simulink model "test_layerwall_static"  (R2013b)
settings: Solver=ode45  StartTime=0.0  StopTime=2*24*3600  RelTol=1e-3
libraries: carnot x9
settings Model: Creator=drhf  LastModifiedBy=drhf
settings OptimizationCC: InlineParams=on

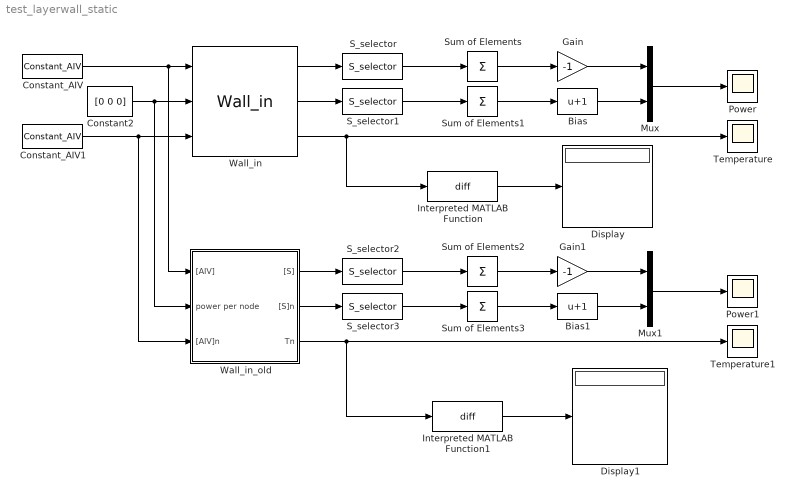
== system test_layerwall_static ==
  Bias : Bias  Bias=1
  Bias1 : Bias  Bias=1
  Constant2 : Constant  Value=[0 0 0]
  Constant_AIV : carnot/Source/Ventilation/Constant_AIV  Tsens=20  Tcon=20  Trad=20  mw=0.012  mco=0.01  rhoair=1.2  cpair=1004  pair=100000  nair=0.5
  Constant_AIV1 : carnot/Source/Ventilation/Constant_AIV  Tsens=0  Tcon=0  Trad=0  mw=0.012  mco=0.01  rhoair=1.2  cpair=1004  pair=100000  nair=0.5
  Display : Display
  Display1 : Display
  Gain : Gain  Gain=-1
  Gain1 : Gain  Gain=-1
  Interpreted MATLAB Function : MATLABFcn  MATLABFcn=diff
  Interpreted MATLAB Function1 : MATLABFcn  MATLABFcn=diff
  Mux : Mux  Inputs=2
  Mux1 : Mux  Inputs=2
  Power : Scope
  Power1 : Scope
      settings: SaveName=ScopeData2
  S_selector{,1..3} (4 alike) : carnot/Outputs/S_selector  e1=off  e2=off  e3=off  e4=off  e5=off  e6=off  e7=on  e8=on  e9=off  e10=off  e11=off  e12=off  e13=off
  Sum of Elements{,1..3} (4 alike) : Sum  Inputs=+
  Temperature : Scope
  Temperature1 : Scope
      settings: SaveName=ScopeData3
  Wall_in : carnot/Load/Houses/wall_floor/Wall_in  wallsize=[10 10]  d=[0.1 0.1 0.1]  cond=[1 1 1]  cwall=[0.28 0.28 0.28]*3600  rho=[2000 200 2000]  emission_in=.96  dactive=[0.075 0.15 0.225]  t0=10  tau=10*3600
  Wall_in_old : Subsystem  AncestorBlock=carnot/Load/Houses/wall_floor/Wall_in  mask(inner wall){wallsize=[10 10], d=[0.1 0.1 0.1], cond=[1 1 1], cwall=[0.28 0.28 0.28]*3600, rho=[2000 200 2000], emission_in=.96, dactive=[0.075 0.15 0.225], t0=10, tau=10*3600}
      mask prompts: wallsize "size of wall [m] [height width]"; d "thickness of layers [m] (vector) (0 = towards this room)"; cond "conductivity of layers [W/(m*K)] (vector)"; cwall "capacity of layers [J/(m³*K)] (vector)"; rho "density of layers [kg/m³]"; emission_in "emission of wall surface"; dactive "depth active layer in m from inner surface  (-1 = none)"; t0 "initial temperature [degree centigrade]"; tau "time-constant of wall [s]"
      mask help:
      | This is the model of an inner wall in a house.
      | first element of the vector = layer to room ([AIV], [S])
      | last element of the vector = layer to neighbour room ([AIV]n, [S]n)
      mask init:
      | position = [0 90 0 ];
      | % nodes = length(d);
      | wallheight = wallsize(1);
      | wallsurface = wallsize(1)*wallsize(2);
      | 
      | if (dactive>=0) 
      |     active = 1;
      | else
      |     active = 0;
      | end
      mask Help: web(fullfile(path_carnot('help'),'Wall_in.html'),'-helpbrowser')
  wires:
  Constant2/1 -> Wall_in_old/2(power per node), Wall_in/2
  Wall_in/1 -> S_selector/1
  Wall_in/2 -> S_selector1/1
  Mux/1 -> Power/1
  Constant_AIV/1 -> Wall_in_old/1("[AIV]"), Wall_in/1
  Constant_AIV1/1 -> Wall_in_old/3("[AIV]n"), Wall_in/3
  S_selector/1 -> Sum of Elements/1
  S_selector1/1 -> Sum of Elements1/1
  Sum of Elements/1 -> Gain/1
  Sum of Elements1/1 -> Bias/1
  Wall_in/3 -> Interpreted MATLAB Function/1, Temperature/1
  Bias/1 -> Mux/2
  Gain/1 -> Mux/1
  Interpreted MATLAB Function/1 -> Display/1
  Wall_in_old/1("[S]") -> S_selector2/1
  Wall_in_old/2("[S]n") -> S_selector3/1
  Mux1/1 -> Power1/1
  S_selector2/1 -> Sum of Elements2/1
  S_selector3/1 -> Sum of Elements3/1
  Sum of Elements2/1 -> Gain1/1
  Sum of Elements3/1 -> Bias1/1
  Wall_in_old/3(Tn) -> Temperature1/1, Interpreted MATLAB Function1/1
  Bias1/1 -> Mux1/2
  Gain1/1 -> Mux1/1
  Interpreted MATLAB Function1/1 -> Display1/1

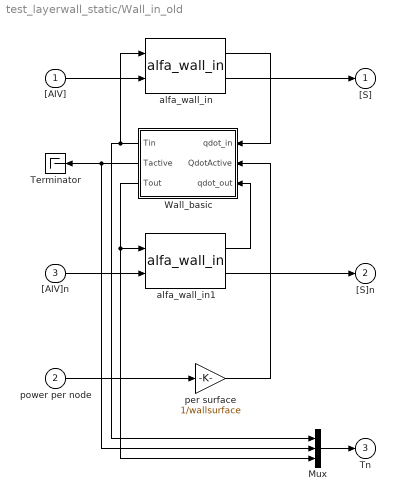
== system test_layerwall_static/Wall_in_old ==
  "[AIV]" : Inport
  power per node : Inport  Port=2
  "[AIV]n" : Inport  Port=3
  Mux : Mux  Inputs=3
  Terminator : Terminator
  Wall_basic : Subsystem  AncestorBlock=carnot/Basic/Thermal_Models/Wall_basic  mask(Wall basic){tau=tau, t0=t0, d=d, dactive=dactive, cond=cond, cwall=cwall, rho=rho}
      mask prompts: tau "Time constant in s"; t0 "Initial temperature in °C"; d "Thickness of layers in m"; dactive "Depth of active layer(s) in m"; cond "Conductivity of layer material in W/m/K"; cwall "Capacity of layer material in J/m³/K"; rho "Density of layer material in kg/m³"
      mask help: Basic model of a wall using a multilayer Beuken model.
      mask Help: web(fullfile(path_carnot('help'),'Wall_basic.html'),'-helpbrowser')
  alfa_wall_in : carnot/Load/Houses/heat_transfer/alfa_wall_in  active=active  emission_in=emission_in  wallsurface=wallsurface
  alfa_wall_in1 : carnot/Load/Houses/heat_transfer/alfa_wall_in  active=active  emission_in=emission_in  wallsurface=wallsurface
  per surface : Gain  Gain=1/wallsurface  SaturateOnIntegerOverflow=on  OutDataTypeStr=Inherit: Same as input  ParamDataTypeStr=Inherit: Same as input
  "[S]" : Outport
  "[S]n" : Outport  Port=2
  Tn : Outport  Port=3
  wires:
  power per node/1 -> per surface/1
  per surface/1 -> Wall_basic/2(QdotActive)
  alfa_wall_in/1 -> Wall_basic/1(qdot_in)
  alfa_wall_in/2 -> "[S]"/1
  Wall_basic/1(Tin) -> Mux/1, alfa_wall_in/1
  "[AIV]"/1 -> alfa_wall_in/2
  alfa_wall_in1/1 -> Wall_basic/3(qdot_out)
  Wall_basic/3(Tout) -> Mux/3, alfa_wall_in1/1
  "[AIV]n"/1 -> alfa_wall_in1/2
  alfa_wall_in1/2 -> "[S]n"/1
  Wall_basic/2(Tactive) -> Mux/2, Terminator/1
  Mux/1 -> Tn/1

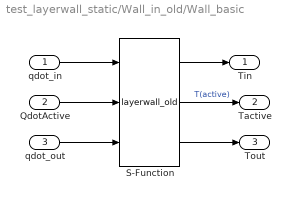
== system test_layerwall_static/Wall_in_old/Wall_basic ==
  qdot_in : Inport
  QdotActive : Inport  Port=2
  qdot_out : Inport  Port=3
  S-Function : S-Function  FunctionName=layerwall_old  Parameters=length(d), tau, t0, d, cond, cwall, rho, length(dactive), dactive  EnableBusSupport=off
  Tin : Outport
  Tactive : Outport  Port=2
  Tout : Outport  Port=3
  wires:
  S-Function/3 -> Tout/1
  qdot_out/1 -> S-Function/3
  S-Function/2 -> Tactive/1  "T(active)"
  QdotActive/1 -> S-Function/2
  S-Function/1 -> Tin/1
  qdot_in/1 -> S-Function/1
